simulink model "CharFu"  (Simulink 5.0)
settings: Solver=ode23tb  StartTime=0.0  StopTime=inf  MaxStep=1/60000  MinStep=1/100000000  RelTol=1e-6
undefined symbols (not defined in the file or in its folder): RFSchar2
libraries: simulink x3, commcontsrc2 x2
settings Model: LastModifiedBy=efst

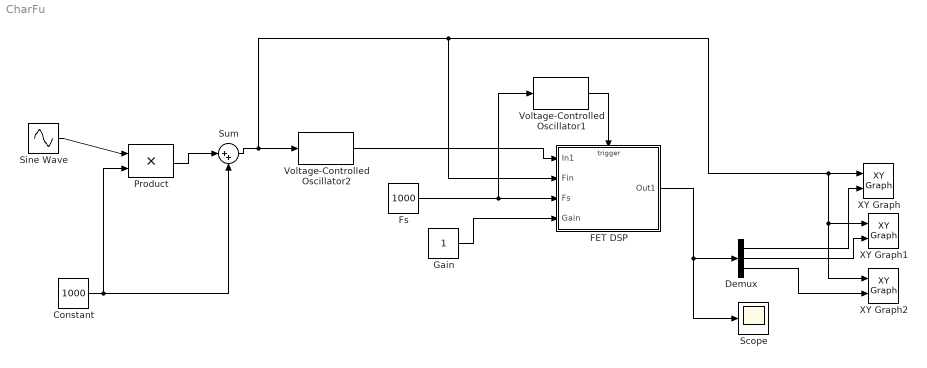
== system CharFu ==
  Constant : Constant  Value=1000
  Demux : Demux  Outputs=3
  FET DSP : Subsystem  TreatAsAtomicUnit=on
  Fs : Constant  Value=1000
  Gain : Constant
  Product : Product  SaturateOnIntegerOverflow=on
  Scope : Scope
      settings: TimeRange=0.3333333333333333  YMin=0  YMax=2000
  Sine Wave : Sin  Frequency=50  SampleTime=0
  Sum : Sum  Inputs=|++  SaturateOnIntegerOverflow=on
  Voltage-Controlled Oscillator1 : commcontsrc2/Voltage-Controlled Oscillator  Ac=1  Fc=0  Kc=1  Ph=0
  Voltage-Controlled Oscillator2 : commcontsrc2/Voltage-Controlled Oscillator  Ac=1  Fc=0  Kc=1  Ph=0
  XY Graph : simulink/Sinks/XY Graph  xmin=0  xmax=3000  ymin=-20  ymax=2000  st=-1
  XY Graph1 : simulink/Sinks/XY Graph  xmin=0  xmax=3000  ymin=-20  ymax=2000  st=-1
  XY Graph2 : simulink/Sinks/XY Graph  xmin=0  xmax=3000  ymin=-20  ymax=2000  st=-1
  wires:
  Fs/1 -> FET DSP/3(Fs), Voltage-Controlled Oscillator1/1
  Gain/1 -> FET DSP/4(Gain)
  Voltage-Controlled Oscillator1/1 -> FET DSP/Trigger
  Sum/1 -> Voltage-Controlled Oscillator2/1, FET DSP/2(Fin), XY Graph/1, XY Graph1/1, XY Graph2/1
  Voltage-Controlled Oscillator2/1 -> FET DSP/1(In1)
  Sine Wave/1 -> Product/1
  Product/1 -> Sum/1
  Constant/1 -> Product/2, Sum/2
  Demux/1 -> XY Graph/2
  Demux/2 -> XY Graph1/2
  Demux/3 -> XY Graph2/2
  FET DSP/1(Out1) -> Demux/1, Scope/1

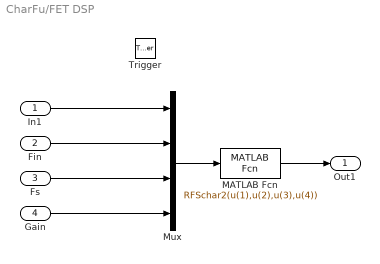
== system CharFu/FET DSP ==
  In1 : Inport
  Fin : Inport  Port=2
  Fs : Inport  Port=3
  Gain : Inport  Port=4
  Trigger : TriggerPort
  MATLAB Fcn : MATLABFcn  MATLABFcn=RFSchar2(u(1),u(2),u(3),u(4))  OutputDimensions=3
  Mux : Mux
  Out1 : Outport
  wires:
  Fin/1 -> Mux/2
  Mux/1 -> MATLAB Fcn/1
  In1/1 -> Mux/1
  MATLAB Fcn/1 -> Out1/1
  Fs/1 -> Mux/3
  Gain/1 -> Mux/4
